simulink model "detectsound"  (R2024b)
settings: Solver=VariableStepAuto  StartTime=0.0  StopTime=20  RelTol=1e-3
libraries: dspvision x8, dspsnks4 x1, deeplib x1, audioai x1
settings Model: Creator=The MathWorks, Inc.  LastModifiedBy=bzhuang
settings DataIOCC: SaveTime=off  ReturnWorkspaceOutputs=off
settings DebuggingCC: UnconnectedInputMsg=warning  UnconnectedOutputMsg=warning  UnconnectedLineMsg=warning
settings ModelReferenceCC: EnableRefExpFcnMdlSchedulingChecks=on
settings RTWCC: GPUComputeCapability=3.5  DLArmComputeVersion=19.05

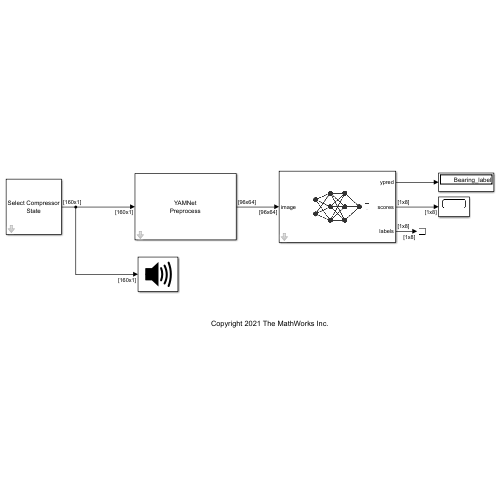
[thumbnail: Simulink's stored preview of the top-level diagram]
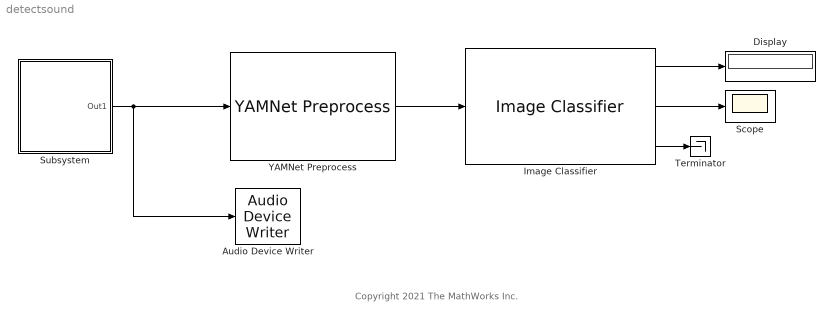
== system detectsound ==
  note: Copyright 2021 The MathWorks Inc.
  Audio Device Writer : dspsnks4/Audio Device Writer  Driver=DirectSound  Device=Default  InheritSampleRate=on  SampleRate=44100  BitDepth=16-bit integer  BufferSize=4096  NumBuffers=10  DefaultOutputChannelMapping=on  OutputChannelMapping=1:2  OutputNumUnderrunSamples=off  DriverIdx=1  DeviceWarnFlag=''
  Display : Display
  Image Classifier : deeplib/Image Classifier  Network=Network from MAT-file  NetworkFunction=squeezenet  NetworkFilePath=airCompressorNet.mat  NetworkClassesVariable=classNames  MiniBatchSize=128  ResizeInput=on  Classification=on  Predictions=on  ForceInterpretedSim=off  PredictMode=All probabilities and labels  K=5
  Scope : Scope
  Subsystem : Subsystem  mask{SoundType=Bearing}
      mask prompts: SoundType "Type"
      mask init:
      | t = get_param(gcb,'SoundType');
      | 
      | val = 1;
      | switch t
      |     case {'Bearing'}
      |         val = 1;
      |     case {'Flywheel'}
      |         val = 2;
      |     case {'Healthy'}
      |         val = 3;
      |     case {'LIV'}
      |         val = 4;
      |     case {'LOV'}
      |         val = 5;
      |     case {'NRV'}
      |         val = 6;
      |     case {'Piston'}
      |         val = 7;
      |     case {'Riderbelt'}
      |         val = 8;
      | end
      | 
      | set_param([gcb '/Constant'],'Value',num2str(val));
      mask TypeOptions SoundType: Bearing | Flywheel | Healthy | LIV | LOV | NRV | Piston | Riderbelt
      mask Display: fprintf('Select Compressor\nState')
  Terminator : Terminator
  YAMNet Preprocess : audioai/YAMNet Preprocess  InputSampleRate=16e3  OverlapPercent=50
  wires:
  Image Classifier/1 -> Display/1
  YAMNet Preprocess/1 -> Image Classifier/1
  Image Classifier/2 -> Scope/1
  Image Classifier/3 -> Terminator/1
  Subsystem/1(Out1) -> Audio Device Writer/1, YAMNet Preprocess/1

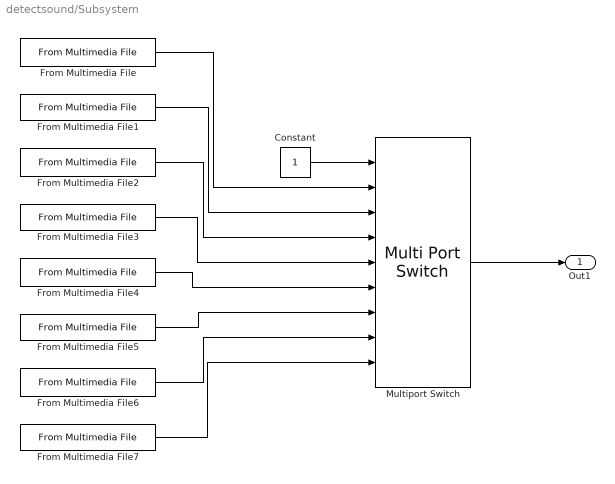
== system detectsound/Subsystem ==
  Constant : Constant
  From Multimedia File : dspvision/From Multimedia File  inputFilename=bearing.wav  readRange=[1 Inf]  loop=on  numPlays=inf  outputStreams=Audio only  videoDataType=single  audioDataType=double  inheritSampleTime=on  userDefinedSampleTime=1/30  noAudioOutput=off  isIntensityVideo=off  fourcc=RGB  colorVideoFormat=Separate color signals  outputEOF=off  dataOrg=Column-major  audioFrameSize=160  computeAudioFrameSize=off  outSamplingMode=Sample based
  From Multimedia File1 : dspvision/From Multimedia File  inputFilename=flywheel.wav  readRange=[1 Inf]  loop=on  numPlays=inf  outputStreams=Audio only  videoDataType=single  audioDataType=double  inheritSampleTime=on  userDefinedSampleTime=1/30  noAudioOutput=off  isIntensityVideo=off  fourcc=RGB  colorVideoFormat=Separate color signals  outputEOF=off  dataOrg=Column-major  audioFrameSize=160  computeAudioFrameSize=off  outSamplingMode=Sample based
  From Multimedia File2 : dspvision/From Multimedia File  inputFilename=healthy.wav  readRange=[1 Inf]  loop=on  numPlays=inf  outputStreams=Audio only  videoDataType=single  audioDataType=double  inheritSampleTime=on  userDefinedSampleTime=1/30  noAudioOutput=off  isIntensityVideo=off  fourcc=RGB  colorVideoFormat=Separate color signals  outputEOF=off  dataOrg=Column-major  audioFrameSize=160  computeAudioFrameSize=off  outSamplingMode=Sample based
  From Multimedia File3 : dspvision/From Multimedia File  inputFilename=liv.wav  readRange=[1 Inf]  loop=on  numPlays=inf  outputStreams=Audio only  videoDataType=single  audioDataType=double  inheritSampleTime=on  userDefinedSampleTime=1/30  noAudioOutput=off  isIntensityVideo=off  fourcc=RGB  colorVideoFormat=Separate color signals  outputEOF=off  dataOrg=Column-major  audioFrameSize=160  computeAudioFrameSize=off  outSamplingMode=Sample based
  From Multimedia File4 : dspvision/From Multimedia File  inputFilename=lov.wav  readRange=[1 Inf]  loop=on  numPlays=inf  outputStreams=Audio only  videoDataType=single  audioDataType=double  inheritSampleTime=on  userDefinedSampleTime=1/30  noAudioOutput=off  isIntensityVideo=off  fourcc=RGB  colorVideoFormat=Separate color signals  outputEOF=off  dataOrg=Column-major  audioFrameSize=160  computeAudioFrameSize=off  outSamplingMode=Sample based
  From Multimedia File5 : dspvision/From Multimedia File  inputFilename=nrv.wav  readRange=[1 Inf]  loop=on  numPlays=inf  outputStreams=Audio only  videoDataType=single  audioDataType=double  inheritSampleTime=on  userDefinedSampleTime=1/30  noAudioOutput=off  isIntensityVideo=off  fourcc=RGB  colorVideoFormat=Separate color signals  outputEOF=off  dataOrg=Column-major  audioFrameSize=160  computeAudioFrameSize=off  outSamplingMode=Sample based
  From Multimedia File6 : dspvision/From Multimedia File  inputFilename=piston.wav  readRange=[1 Inf]  loop=on  numPlays=inf  outputStreams=Audio only  videoDataType=single  audioDataType=double  inheritSampleTime=on  userDefinedSampleTime=1/30  noAudioOutput=off  isIntensityVideo=off  fourcc=RGB  colorVideoFormat=Separate color signals  outputEOF=off  dataOrg=Column-major  audioFrameSize=160  computeAudioFrameSize=off  outSamplingMode=Sample based
  From Multimedia File7 : dspvision/From Multimedia File  inputFilename=riderbelt.wav  readRange=[1 Inf]  loop=on  numPlays=inf  outputStreams=Audio only  videoDataType=single  audioDataType=double  inheritSampleTime=on  userDefinedSampleTime=1/30  noAudioOutput=off  isIntensityVideo=off  fourcc=RGB  colorVideoFormat=Separate color signals  outputEOF=off  dataOrg=Column-major  audioFrameSize=160  computeAudioFrameSize=off  outSamplingMode=Sample based
  Multiport Switch : MultiPortSwitch  Inputs=8  SaturateOnIntegerOverflow=off  InputSameDT=off
  Out1 : Outport
  wires:
  From Multimedia File2/1 -> Multiport Switch/4
  From Multimedia File/1 -> Multiport Switch/2
  From Multimedia File6/1 -> Multiport Switch/8
  From Multimedia File3/1 -> Multiport Switch/5
  From Multimedia File4/1 -> Multiport Switch/6
  From Multimedia File1/1 -> Multiport Switch/3
  From Multimedia File5/1 -> Multiport Switch/7
  From Multimedia File7/1 -> Multiport Switch/9
  Constant/1 -> Multiport Switch/1
  Multiport Switch/1 -> Out1/1
